simulink model "NetworkUDPReceive1NSP"  (R2016b)
settings: Solver=FixedStepDiscrete  StartTime=0.0  StopTime=inf  FixedStep=sCoreParams.core.stepPeriod  RelTol=1e-3
undefined symbols (not defined in the file or in its folder): sCoreParams
libraries: slrtlib x4, dspsigattribs x2, xpcrtudplib x2
settings Model: xpc_rtwmakecfg_data=_xpcetherlib__xpcether8255xlib__xpcetherGbElib__xpciplib__xpcnblib_  Creator=anish  LastModifiedBy=Rack_Trois
settings SolverCC: EnableConcurrentExecution=on
settings DataIOCC: LimitDataPoints=on  SaveFormat=StructureWithTime  SignalLoggingSaveFormat=ModelDataLogs
settings OptimizationCC: BlockReduction=off  DefaultParameterBehavior=Inlined  OptimizeBlockIOStorage=off  BufferReuse=off  GlobalBufferReuse=off  ExpressionFolding=off  LocalBlockOutputs=off  LifeSpan=inf
settings DebuggingCC: SaveWithParameterizedLinksMsg=none  MultiTaskDSMMsg=warning  MultiTaskCondExecSysMsg=none  StateNameClashWarn=warning  SFUnexpectedBacktrackingDiag=warning  SFNoUnconditionalDefaultTransitionDiag=warning  SFExecutionAtInitializationDiag=none
settings HardwareCC: ProdBitPerPointer=32  ProdBitPerSizeT=32  ProdBitPerPtrDiffT=32  ProdLargestAtomicFloat=None  ProdWordSize=32  ProdLongLongMode=on  ProdHWDeviceType=Generic->32-bit x86 compatible
settings ModelReferenceCC: EnableRefExpFcnMdlSchedulingChecks=off  ModelReferenceNumInstancesAllowed=Single  ModelReferencePassRootInputsByReference=off
settings RTWCC: SystemTargetFile=slrt.tlc  TemplateMakefile=slrt_default_tmf  Description=Simulink Real-Time  RTWCompilerOptimization=on
settings ConfigComp: CovMetricSettings=dw  CovHtmlReporting=on  CovSaveCumulativeToWorkspaceVar=on  CovSaveSingleToWorkspaceVar=on  CovExternalEMLEnable=off

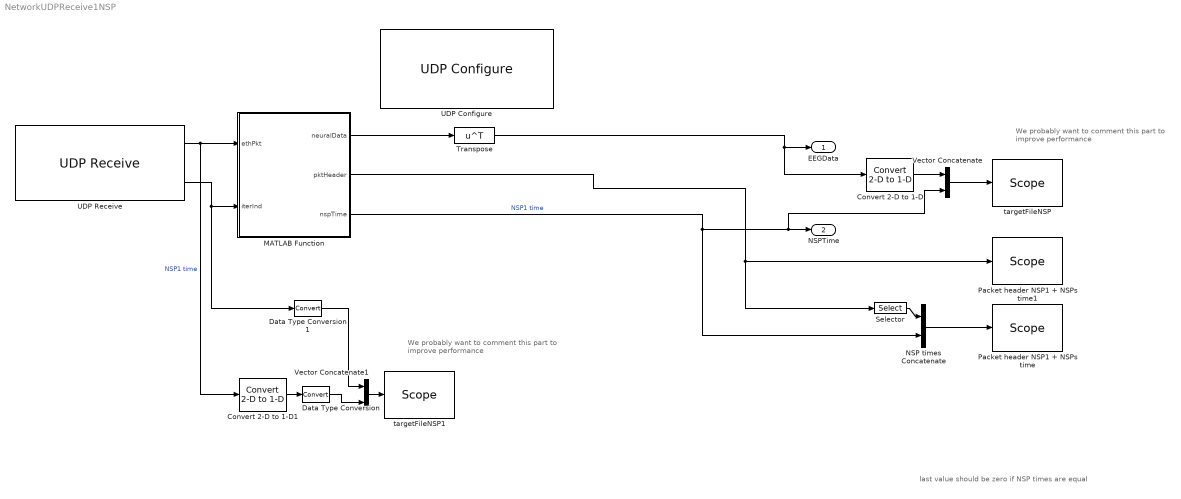
== system NetworkUDPReceive1NSP ==
  note: We probably want to comment this part
      | to improve performance
  note: last value should be zero if NSP times are equal
  note: We probably want to comment this part
      | to improve performance
  Convert 2-D to 1-D : dspsigattribs/Convert 2-D to 1-D
  Convert 2-D to 1-D1 : dspsigattribs/Convert 2-D to 1-D
  Data Type Conversion : DataTypeConversion
  Data Type Conversion1 : DataTypeConversion
  MATLAB Function : MATLAB Function  TreatAsAtomicUnit=on
  NSP times Concatenate : Concatenate
  Packet header NSP1 + NSPs time : slrtlib/Displays and Logging/Scope   scopeno=11  scopetype=Target  autostart=on  viewmode=Numerical  formatstr='%15.6f'  grid=on  ylimits=[0,0]  nosamples=100  noprepostsamples=0  interleave=1  triggermode=FreeRun  triggersignal=1  trigsignalfromport=off  triggerlevel=0.0  triggerslope=Either  triggerscope=1  triggersample=0  filename=data.dat  mode=Lazy  writesize=512  autorestart=off  dynamicfilemode=off  maxwritefilesize=512*1024^2
  Packet header NSP1 + NSPs time1 : slrtlib/Displays and Logging/Scope   scopeno=1  scopetype=Target  autostart=on  viewmode=Numerical  formatstr='%15.6f'  grid=on  ylimits=[0,0]  nosamples=1000  noprepostsamples=0  interleave=1  triggermode=FreeRun  triggersignal=1  trigsignalfromport=off  triggerlevel=0.0  triggerslope=Either  triggerscope=1  triggersample=0  filename=data.dat  mode=Lazy  writesize=512  autorestart=off  dynamicfilemode=off  maxwritefilesize=512*1024^2
  Selector : Selector  InputPortWidth=13  IndexOptions=Index vector (dialog)  Indices=[9:13]  OutputSizes=1
  Transpose : Math  Operator=transpose  SaturateOnIntegerOverflow=on
  UDP Configure : xpcrtudplib/UDP Configure  Priority=-1  IpAddress=192.168.137.7  SubnetMask=255.255.255.0  Gateway=0.0.0.0  PciBus=sCoreParams.network.pciBus(1)  PciSlot=sCoreParams.network.pciSlot(1)  ID=1  tune=0
  UDP Receive : xpcrtudplib/UDP Receive  ipAddressVal=192.168.137.7  localPort=51002  rcvWidth=2048  rcvFmAny=on  fmAddress=0.0.0.0  sampleTime=sCoreParams.core.stepPeriod
  Vector Concatenate : Concatenate
  Vector Concatenate1 : Concatenate
  targetFileNSP : slrtlib/Displays and Logging/Scope   scopeno=10  scopetype=File  autostart=on  viewmode=Numerical  formatstr='%15.6f'  grid=on  ylimits=[0,0]  nosamples=1000  noprepostsamples=0  interleave=1  triggermode=FreeRun  triggersignal=1  trigsignalfromport=off  triggerlevel=0.0  triggerslope=Either  triggerscope=1  triggersample=0  filename=NSP1<%%%>.dat  mode=Lazy  writesize=512  autorestart=on  dynamicfilemode=on  maxwritefilesize=512*1024^2
  targetFileNSP1 : slrtlib/Displays and Logging/Scope   scopeno=12  scopetype=File  autostart=on  viewmode=Numerical  formatstr='%15.6f'  grid=on  ylimits=[0,0]  nosamples=1000  noprepostsamples=0  interleave=1  triggermode=FreeRun  triggersignal=1  trigsignalfromport=off  triggerlevel=0.0  triggerslope=Either  triggerscope=1  triggersample=0  filename=ETH_<%%%>.dat  mode=Commit  writesize=512  autorestart=on  dynamicfilemode=on  maxwritefilesize=512*1024^2
  EEGData : Outport  PortDimensions=[sCoreParams.core.samplesPerStep sCoreParams.core.maxChannelsPerNSP]  SampleTime=sCoreParams.core.stepPeriod
  NSPTime : Outport  Port=2
  wires:
  MATLAB Function/2(pktHeader) -> Selector/1, Packet header NSP1 + NSPs time1/1
  MATLAB Function/3(nspTime) -> NSP times Concatenate/2, Vector Concatenate/2, NSPTime/1  "NSP1 time"
  Transpose/1 -> EEGData/1, Convert 2-D to 1-D/1
  NSP times Concatenate/1 -> Packet header NSP1 + NSPs time/1
  Convert 2-D to 1-D/1 -> Vector Concatenate/1
  Vector Concatenate/1 -> targetFileNSP/1
  MATLAB Function/1(neuralData) -> Transpose/1
  UDP Receive/2 -> Data Type Conversion1/1, MATLAB Function/2(iterInd)
  UDP Receive/1 -> MATLAB Function/1(ethPkt), Convert 2-D to 1-D1/1  "NSP1 time"
  Convert 2-D to 1-D1/1 -> Data Type Conversion/1
  Selector/1 -> NSP times Concatenate/1
  Vector Concatenate1/1 -> targetFileNSP1/1
  Data Type Conversion/1 -> Vector Concatenate1/2
  Data Type Conversion1/1 -> Vector Concatenate1/1

== matlab function NetworkUDPReceive1NSP/MATLAB Function ==
  data: ethPkt input; neuralData output; iterInd input; pktHeader output; nspTime output
function [neuralData,pktHeader,nspTime]  = PacketParser(ethPkt,iterInd)
%#codegen

%[neuralData,spikeCounts,spikeTimes,pktHeader,nspTime] = PacketParser_EML(ethPkt,iterInd);
newAcquisition=0; % See if we need to change it when starting new block  
nspTime =0;

[neuralData,pktHeader,nspTime] = PacketParserBlackRock_EML(ethPkt,newAcquisition);
